simulink model "Filter_cascade"  (R2020a)
settings: Solver=FixedStepAuto  StartTime=0.0  StopTime=10.0  FixedStep=0.1  RelTol=1e-3
settings Model: Creator=Anjali123  LastModifiedBy=Anjali123
settings DataIOCC: SaveOutput=off  SaveTime=off

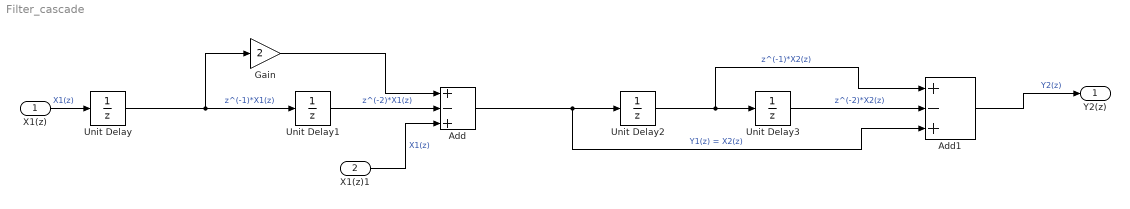
== system Filter_cascade ==
  X1(z) : Inport  OutDataTypeStr=double  PortDimensions=1  SampleTime=[0.10000000000000001,0]
  X1(z)1 : Inport  Port=2  OutDataTypeStr=double  PortDimensions=1  SampleTime=[0.10000000000000001,0]
  Add : Sum  Inputs=+-+
  Add1 : Sum  Inputs=+-+
  Gain : Gain  Gain=2
  Unit Delay{,1..3} (4 alike) : UnitDelay  SampleTime=-1  HasFrameUpgradeWarning=on
  Y2(z) : Outport  OutDataTypeStr=double  PortDimensions=1  SampleTime=[0.10000000000000001,0]
  wires:
  Add1/1 -> Y2(z)/1  "Y2(z)"
  Unit Delay2/1 -> Unit Delay3/1, Add1/1  "z^(-1)*X2(z)"
  Unit Delay1/1 -> Add/2  "z^(-2)*X1(z)"
  Add/1 -> Unit Delay2/1, Add1/3  "Y1(z) = X2(z)"
  Unit Delay/1 -> Unit Delay1/1, Gain/1  "z^(-1)*X1(z)"
  X1(z)1/1 -> Add/3  "X1(z)"
  Gain/1 -> Add/1
  X1(z)/1 -> Unit Delay/1  "X1(z)"
  Unit Delay3/1 -> Add1/2  "z^(-2)*X2(z)"
